simulink model "ussie_da_sdet"  (Simulink 6.4)
settings: Solver=ode45  StartTime=0.0  StopTime=10.0  RelTol=1e-3
libraries: vipsnks x2, vipconversions x1, imaqlib x1
settings Model: LastModifiedBy=Raza

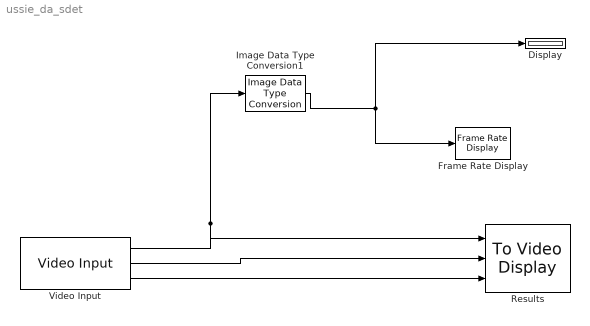
== system ussie_da_sdet ==
  Display : Display
  Frame Rate Display : vipsnks/Frame Rate Display  DialogController=vipDDGCreate  DialogControllerArgs=DataTag0  UpdateRate=1
  Image Data Type Conversion1 : vipconversions/Image Data Type Conversion  outDT=double  isSigned=on  wordLen=16  numFracBits=0
  Results : vipsnks/To Video Display  inputType=RGB  OutputDevice=On-screen video monitor  fullScreen=off  videoWindowX=39  videoWindowY=82  saveWindowSize=off  videoWindowWidth=776  videoWindowHeight=603
  Video Input : imaqlib/Video Input  DialogController=imaqcreatedialog  DialogControllerArgs=DataTag1  VideoDeviceMenu=1 (Bt878 TV Card)  VideoDevice=1 (Bt878 TV Card)  VideoStreamFormatMenu=RGB555_768x576  VideoStreamFormat=RGB555_768x576  VideoFrameSize=INPUTSIZE  FrameRate=30 fps  DataType=uint8
  wires:
  Video Input/1 -> Image Data Type Conversion1/1, Results/1
  Video Input/2 -> Results/2
  Video Input/3 -> Results/3
  Image Data Type Conversion1/1 -> Display/1, Frame Rate Display/1
